simulink model "mariner_NNcont"  (R2018b)
settings: Solver=FixedStepAuto  StartTime=0.0  StopTime=600  FixedStep=0.1  RelTol=1e-3
libraries: neural x50, simulink x1
(part 2 of 2)

== system mariner_NNcont/Controller/NN controller (w.o process) 2 inputs/Layer 3/LW{3,2} ==
  "ad{3,2}" : Inport  PortDimensions=10
      mask Display: e = 0.06;c1 = [120 230 180]/255;c2 = ([120 230 180]+0)/(256+128);c3 = ([120 230 180]+128)/(256+128);patch([0 1 1 0],[0 0 1 1],c1);patch([0 1 1 1-e 1-e 0+e],[0 0 1 1-e 0+e 0+e],c2);patch([0 0 1 1-e 0+e 0+e],[0 1 1 1-e 1-e 0+e],c3);plot([0 1 1 0 0],[0 0 1 1 0]);
  "IW{3,2}(1,:)'" : Constant  Value=[-0.48696402852144660133859588313498534262180328369140625;-0.84681627945538029411665092993644066154956817626953125;0;0;1.0152212048569406732667630421929061412811279296875;0;0;0.89789896717366257661296913283877074718475341796875;0.1672600396616808204885984423526679165661334991455078125;0]
      mask Display: e = 0.06;c1 = [120 150 230]/255;c2 = ([120 150 230]+0)/383;c3 = ([120 150 230]+128)/383;patch([0 1 1 0],[0 0 1 1],c1);patch([0 1 1 1-e 1-e 0+e],[0 0 1 1-e 0+e 0+e],c2);patch([0 0 1 1-e 0+e 0+e],[0 1 1 1-e 1-e 0+e],c3);plot([0 1 1 0 0],[0 0 1 1 0]);disp('weights');
  Mux : Mux  Inputs=1
      mask Display: e = 0.06;c1 = [120 150 230]/255;c2 = ([120 150 230]+0)/383;c3 = ([120 150 230]+128)/383;patch([0 1 1 0],[0 0 1 1],c1);patch([0 1 1 1-e 1-e 0+e],[0 0 1 1-e 0+e 0+e],c2);patch([0 0 1 1-e 0+e 0+e],[0 1 1 1-e 1-e 0+e],c3);plot([0 1 1 0 0],[0 0 1 1 0]);disp('Mux');
  dotprod1 : neural/Weight Functions/dotprod
  "lz{3,2}" : Outport
      mask Display: e = 0.06;c1 = [120 230 180]/255;c2 = ([120 230 180]+0)/(256+128);c3 = ([120 230 180]+128)/(256+128);patch([0 1 1 0],[0 0 1 1],c1);patch([0 1 1 1-e 1-e 0+e],[0 0 1 1-e 0+e 0+e],c2);patch([0 0 1 1-e 0+e 0+e],[0 1 1 1-e 1-e 0+e],c3);plot([0 1 1 0 0],[0 0 1 1 0]);
  wires:
  Mux/1 -> "lz{3,2}"/1
  dotprod1/1 -> Mux/1
  "ad{3,2}"/1 -> dotprod1/2
  "IW{3,2}(1,:)'"/1 -> dotprod1/1

== system mariner_NNcont/Controller/NN controller (w//o process) 3 inputs/Layer 1/Delays 1 ==
  "p{1}" : Inport  PortDimensions=3
      mask Display: e = 0.06;c1 = [120 230 180]/255;c2 = ([120 230 180]+0)/(256+128);c3 = ([120 230 180]+128)/(256+128);patch([0 1 1 0],[0 0 1 1],c1);patch([0 1 1 1-e 1-e 0+e],[0 0 1 1-e 0+e 0+e],c2);patch([0 0 1 1-e 0+e 0+e],[0 1 1 1-e 1-e 0+e],c3);plot([0 1 1 0 0],[0 0 1 1 0]);
  mux : Mux  Inputs=1
      mask Display: e = 0.06;c1 = [120 150 230]/255;c2 = ([120 150 230]+0)/383;c3 = ([120 150 230]+128)/383;patch([0 1 1 0],[0 0 1 1],c1);patch([0 1 1 1-e 1-e 0+e],[0 0 1 1-e 0+e 0+e],c2);patch([0 0 1 1-e 0+e 0+e],[0 1 1 1-e 1-e 0+e],c3);plot([0 1 1 0 0],[0 0 1 1 0]);disp('Mux')
  "pd{1,1}" : Outport
      mask Display: e = 0.06;c1 = [120 230 180]/255;c2 = ([120 230 180]+0)/(256+128);c3 = ([120 230 180]+128)/(256+128);patch([0 1 1 0],[0 0 1 1],c1);patch([0 1 1 1-e 1-e 0+e],[0 0 1 1-e 0+e 0+e],c2);patch([0 0 1 1-e 0+e 0+e],[0 1 1 1-e 1-e 0+e],c3);plot([0 1 1 0 0],[0 0 1 1 0]);
  wires:
  mux/1 -> "pd{1,1}"/1
  "p{1}"/1 -> mux/1

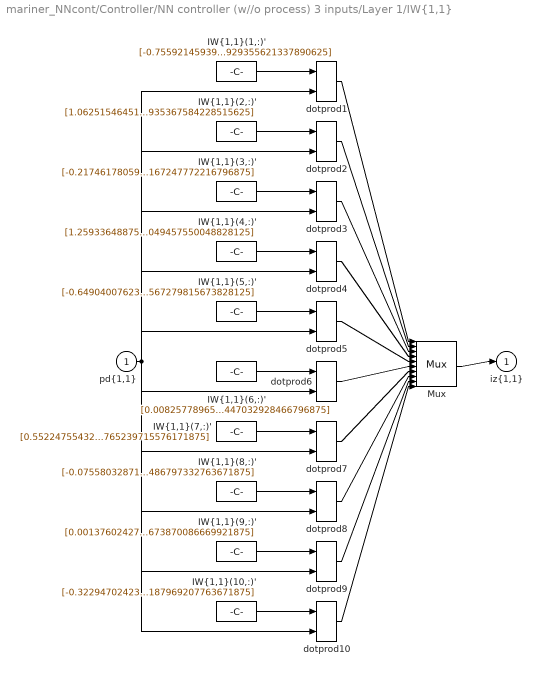
== system mariner_NNcont/Controller/NN controller (w//o process) 3 inputs/Layer 1/IW{1,1} ==
  "pd{1,1}" : Inport  PortDimensions=3
      mask Display: e = 0.06;c1 = [120 230 180]/255;c2 = ([120 230 180]+0)/(256+128);c3 = ([120 230 180]+128)/(256+128);patch([0 1 1 0],[0 0 1 1],c1);patch([0 1 1 1-e 1-e 0+e],[0 0 1 1-e 0+e 0+e],c2);patch([0 0 1 1-e 0+e 0+e],[0 1 1 1-e 1-e 0+e],c3);plot([0 1 1 0 0],[0 0 1 1 0]);
  "IW{1,1}(1,:)'" : Constant  Value=[-0.7559214593946765869958426264929585158824920654296875;-0.0246645007907288528470335364772836328484117984771728515625;0.031250654238925125449899411478327238000929355621337890625]
      mask Display: e = 0.06;c1 = [120 150 230]/255;c2 = ([120 150 230]+0)/383;c3 = ([120 150 230]+128)/383;patch([0 1 1 0],[0 0 1 1],c1);patch([0 1 1 1-e 1-e 0+e],[0 0 1 1-e 0+e 0+e],c2);patch([0 0 1 1-e 0+e 0+e],[0 1 1 1-e 1-e 0+e],c3);plot([0 1 1 0 0],[0 0 1 1 0]);disp('Weights');
  "IW{1,1}(10,:)'" : Constant  Value=[-0.32294702423027465965077453802223317325115203857421875;-0.1071172496029534626504897687482298351824283599853515625;0.0984226273448558230949601011161576025187969207763671875]
      mask Display: e = 0.06;c1 = [120 150 230]/255;c2 = ([120 150 230]+0)/383;c3 = ([120 150 230]+128)/383;patch([0 1 1 0],[0 0 1 1],c1);patch([0 1 1 1-e 1-e 0+e],[0 0 1 1-e 0+e 0+e],c2);patch([0 0 1 1-e 0+e 0+e],[0 1 1 1-e 1-e 0+e],c3);plot([0 1 1 0 0],[0 0 1 1 0]);disp('Weights');
  "IW{1,1}(2,:)'" : Constant  Value=[1.0625154645189052171616594932856969535350799560546875;0.1231458876428332960273337448597885668277740478515625;-0.12089326066373841384038456681082607246935367584228515625]
      mask Display: e = 0.06;c1 = [120 150 230]/255;c2 = ([120 150 230]+0)/383;c3 = ([120 150 230]+128)/383;patch([0 1 1 0],[0 0 1 1],c1);patch([0 1 1 1-e 1-e 0+e],[0 0 1 1-e 0+e 0+e],c2);patch([0 0 1 1-e 0+e 0+e],[0 1 1 1-e 1-e 0+e],c3);plot([0 1 1 0 0],[0 0 1 1 0]);disp('Weights');
  "IW{1,1}(3,:)'" : Constant  Value=[-0.2174617805911333856538902864485862664878368377685546875;-0.05222802197034777382800285749908653087913990020751953125;0.0405135495877011198029293836953002028167247772216796875]
      mask Display: e = 0.06;c1 = [120 150 230]/255;c2 = ([120 150 230]+0)/383;c3 = ([120 150 230]+128)/383;patch([0 1 1 0],[0 0 1 1],c1);patch([0 1 1 1-e 1-e 0+e],[0 0 1 1-e 0+e 0+e],c2);patch([0 0 1 1-e 0+e 0+e],[0 1 1 1-e 1-e 0+e],c3);plot([0 1 1 0 0],[0 0 1 1 0]);disp('Weights');
  "IW{1,1}(4,:)'" : Constant  Value=[1.259336488753712846033749883645214140415191650390625;0.12858048113142583890322612205636687576770782470703125;-0.12856053982931670010003699644585140049457550048828125]
      mask Display: e = 0.06;c1 = [120 150 230]/255;c2 = ([120 150 230]+0)/383;c3 = ([120 150 230]+128)/383;patch([0 1 1 0],[0 0 1 1],c1);patch([0 1 1 1-e 1-e 0+e],[0 0 1 1-e 0+e 0+e],c2);patch([0 0 1 1-e 0+e 0+e],[0 1 1 1-e 1-e 0+e],c3);plot([0 1 1 0 0],[0 0 1 1 0]);disp('Weights');
  "IW{1,1}(5,:)'" : Constant  Value=[-0.64904007623710613383849477031617425382137298583984375;-0.07309425860026873278396664090905687771737575531005859375;0.07976020263064671766972679733953555114567279815673828125]
      mask Display: e = 0.06;c1 = [120 150 230]/255;c2 = ([120 150 230]+0)/383;c3 = ([120 150 230]+128)/383;patch([0 1 1 0],[0 0 1 1],c1);patch([0 1 1 1-e 1-e 0+e],[0 0 1 1-e 0+e 0+e],c2);patch([0 0 1 1-e 0+e 0+e],[0 1 1 1-e 1-e 0+e],c3);plot([0 1 1 0 0],[0 0 1 1 0]);disp('Weights');
  "IW{1,1}(6,:)'" : Constant  Value=[0.0082577896598646817472033632157035754062235355377197265625;-0.043198240899638508383251433997429558075964450836181640625;0.038175683250024732007243954967634635977447032928466796875]
      mask Display: e = 0.06;c1 = [120 150 230]/255;c2 = ([120 150 230]+0)/383;c3 = ([120 150 230]+128)/383;patch([0 1 1 0],[0 0 1 1],c1);patch([0 1 1 1-e 1-e 0+e],[0 0 1 1-e 0+e 0+e],c2);patch([0 0 1 1-e 0+e 0+e],[0 1 1 1-e 1-e 0+e],c3);plot([0 1 1 0 0],[0 0 1 1 0]);disp('Weights');
  "IW{1,1}(7,:)'" : Constant  Value=[0.5522475543267157949145484963082708418369293212890625;0.038102250776124939324329687906356411986052989959716796875;-0.034686212621672755929136400254719774238765239715576171875]
      mask Display: e = 0.06;c1 = [120 150 230]/255;c2 = ([120 150 230]+0)/383;c3 = ([120 150 230]+128)/383;patch([0 1 1 0],[0 0 1 1],c1);patch([0 1 1 1-e 1-e 0+e],[0 0 1 1-e 0+e 0+e],c2);patch([0 0 1 1-e 0+e 0+e],[0 1 1 1-e 1-e 0+e],c3);plot([0 1 1 0 0],[0 0 1 1 0]);disp('Weights');
  "IW{1,1}(8,:)'" : Constant  Value=[-0.075580328717062272847471149361808784306049346923828125;-0.1184719143490288451037173445001826621592044830322265625;0.09404446170240236824167112672512303106486797332763671875]
      mask Display: e = 0.06;c1 = [120 150 230]/255;c2 = ([120 150 230]+0)/383;c3 = ([120 150 230]+128)/383;patch([0 1 1 0],[0 0 1 1],c1);patch([0 1 1 1-e 1-e 0+e],[0 0 1 1-e 0+e 0+e],c2);patch([0 0 1 1-e 0+e 0+e],[0 1 1 1-e 1-e 0+e],c3);plot([0 1 1 0 0],[0 0 1 1 0]);disp('Weights');
  "IW{1,1}(9,:)'" : Constant  Value=[0.0013760242756342658428103664647323967074044048786163330078125;-0.00880586545902399542296024037568713538348674774169921875;-0.0023602613359520771378619041769297837163321673870086669921875]
      mask Display: e = 0.06;c1 = [120 150 230]/255;c2 = ([120 150 230]+0)/383;c3 = ([120 150 230]+128)/383;patch([0 1 1 0],[0 0 1 1],c1);patch([0 1 1 1-e 1-e 0+e],[0 0 1 1-e 0+e 0+e],c2);patch([0 0 1 1-e 0+e 0+e],[0 1 1 1-e 1-e 0+e],c3);plot([0 1 1 0 0],[0 0 1 1 0]);disp('Weights');
  Mux : Mux  Inputs=10
      mask Display: e = 0.06;c1 = [120 150 230]/255;c2 = ([120 150 230]+0)/383;c3 = ([120 150 230]+128)/383;patch([0 1 1 0],[0 0 1 1],c1);patch([0 1 1 1-e 1-e 0+e],[0 0 1 1-e 0+e 0+e],c2);patch([0 0 1 1-e 0+e 0+e],[0 1 1 1-e 1-e 0+e],c3);plot([0 1 1 0 0],[0 0 1 1 0]);disp('Mux');
  dotprod{1..10} (10 alike) : neural/Weight Functions/dotprod
  "iz{1,1}" : Outport
      mask Display: e = 0.06;c1 = [120 230 180]/255;c2 = ([120 230 180]+0)/(256+128);c3 = ([120 230 180]+128)/(256+128);patch([0 1 1 0],[0 0 1 1],c1);patch([0 1 1 1-e 1-e 0+e],[0 0 1 1-e 0+e 0+e],c2);patch([0 0 1 1-e 0+e 0+e],[0 1 1 1-e 1-e 0+e],c3);plot([0 1 1 0 0],[0 0 1 1 0]);
  wires:
  Mux/1 -> "iz{1,1}"/1
  dotprod10/1 -> Mux/10
  "IW{1,1}(10,:)'"/1 -> dotprod10/1
  dotprod9/1 -> Mux/9
  "IW{1,1}(9,:)'"/1 -> dotprod9/1
  dotprod8/1 -> Mux/8
  "IW{1,1}(8,:)'"/1 -> dotprod8/1
  dotprod7/1 -> Mux/7
  "IW{1,1}(7,:)'"/1 -> dotprod7/1
  dotprod6/1 -> Mux/6
  "IW{1,1}(6,:)'"/1 -> dotprod6/1
  dotprod5/1 -> Mux/5
  "IW{1,1}(5,:)'"/1 -> dotprod5/1
  dotprod4/1 -> Mux/4
  "IW{1,1}(4,:)'"/1 -> dotprod4/1
  dotprod3/1 -> Mux/3
  "IW{1,1}(3,:)'"/1 -> dotprod3/1
  dotprod2/1 -> Mux/2
  "IW{1,1}(2,:)'"/1 -> dotprod2/1
  dotprod1/1 -> Mux/1
  "pd{1,1}"/1 -> dotprod10/2, dotprod9/2, dotprod8/2, dotprod7/2, dotprod6/2, dotprod5/2, dotprod4/2, dotprod3/2, dotprod2/2, dotprod1/2
  "IW{1,1}(1,:)'"/1 -> dotprod1/1

== system mariner_NNcont/Controller/NN controller (w//o process) 3 inputs/Layer 2/Delays 1 ==
  "p{2}" : Inport  PortDimensions=10
      mask Display: e = 0.06;c1 = [120 230 180]/255;c2 = ([120 230 180]+0)/(256+128);c3 = ([120 230 180]+128)/(256+128);patch([0 1 1 0],[0 0 1 1],c1);patch([0 1 1 1-e 1-e 0+e],[0 0 1 1-e 0+e 0+e],c2);patch([0 0 1 1-e 0+e 0+e],[0 1 1 1-e 1-e 0+e],c3);plot([0 1 1 0 0],[0 0 1 1 0]);
  mux : Mux  Inputs=1
      mask Display: e = 0.06;c1 = [120 150 230]/255;c2 = ([120 150 230]+0)/383;c3 = ([120 150 230]+128)/383;patch([0 1 1 0],[0 0 1 1],c1);patch([0 1 1 1-e 1-e 0+e],[0 0 1 1-e 0+e 0+e],c2);patch([0 0 1 1-e 0+e 0+e],[0 1 1 1-e 1-e 0+e],c3);plot([0 1 1 0 0],[0 0 1 1 0]);disp('Mux')
  "pd{2,1}" : Outport
      mask Display: e = 0.06;c1 = [120 230 180]/255;c2 = ([120 230 180]+0)/(256+128);c3 = ([120 230 180]+128)/(256+128);patch([0 1 1 0],[0 0 1 1],c1);patch([0 1 1 1-e 1-e 0+e],[0 0 1 1-e 0+e 0+e],c2);patch([0 0 1 1-e 0+e 0+e],[0 1 1 1-e 1-e 0+e],c3);plot([0 1 1 0 0],[0 0 1 1 0]);
  wires:
  mux/1 -> "pd{2,1}"/1
  "p{2}"/1 -> mux/1

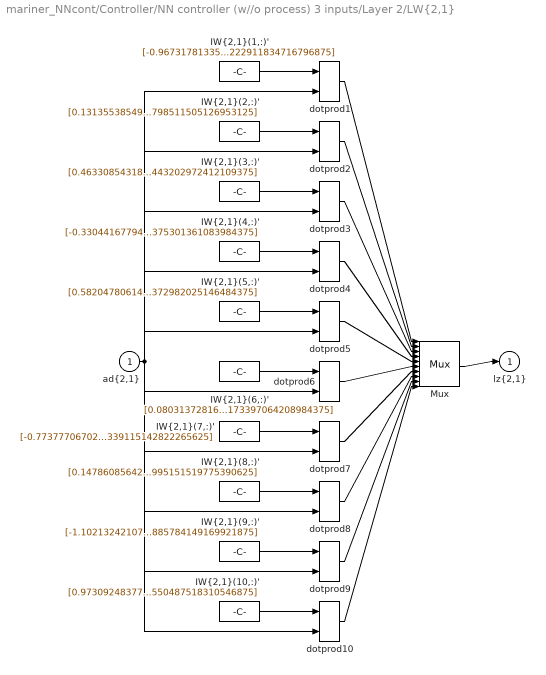
== system mariner_NNcont/Controller/NN controller (w//o process) 3 inputs/Layer 2/LW{2,1} ==
  "ad{2,1}" : Inport  PortDimensions=10
      mask Display: e = 0.06;c1 = [120 230 180]/255;c2 = ([120 230 180]+0)/(256+128);c3 = ([120 230 180]+128)/(256+128);patch([0 1 1 0],[0 0 1 1],c1);patch([0 1 1 1-e 1-e 0+e],[0 0 1 1-e 0+e 0+e],c2);patch([0 0 1 1-e 0+e 0+e],[0 1 1 1-e 1-e 0+e],c3);plot([0 1 1 0 0],[0 0 1 1 0]);
  "IW{2,1}(1,:)'" : Constant  Value=[-0.9673178133559503510952026772429235279560089111328125;0.53839778171147634200366383083746768534183502197265625;-0.722317642025362971480717533268034458160400390625;0.8553552777126747219682556533371098339557647705078125;0.275878338813815293661946270731277763843536376953125;-0.02755546810020788328632335151269217021763324737548828125;0.82237984032601907369297578043187968432903289794921875;-0.2547472202517508943486745920381508767604827880859375;-0.61557536337765605960470338686718605458736419677734375;0.153664159931131638625600999148446135222911834716796875]
      mask Display: e = 0.06;c1 = [120 150 230]/255;c2 = ([120 150 230]+0)/383;c3 = ([120 150 230]+128)/383;patch([0 1 1 0],[0 0 1 1],c1);patch([0 1 1 1-e 1-e 0+e],[0 0 1 1-e 0+e 0+e],c2);patch([0 0 1 1-e 0+e 0+e],[0 1 1 1-e 1-e 0+e],c3);plot([0 1 1 0 0],[0 0 1 1 0]);disp('weights');
  "IW{2,1}(10,:)'" : Constant  Value=[0.97309248377746315750158601076691411435604095458984375;-0.845856659992735959718856975086964666843414306640625;0.0295346903368784718946216116819414310157299041748046875;-1.1110911960074727478087197596323676407337188720703125;0.3060928624502607942048371114651672542095184326171875;-0.026387217399169611564690995919590932317078113555908203125;-0.554579983764879269614311851910315454006195068359375;-0.7959887047101454893294203429832123219966888427734375;-0.53675247865637409905303911727969534695148468017578125;-0.30786197281541471948429489202680997550487518310546875]
      mask Display: e = 0.06;c1 = [120 150 230]/255;c2 = ([120 150 230]+0)/383;c3 = ([120 150 230]+128)/383;patch([0 1 1 0],[0 0 1 1],c1);patch([0 1 1 1-e 1-e 0+e],[0 0 1 1-e 0+e 0+e],c2);patch([0 0 1 1-e 0+e 0+e],[0 1 1 1-e 1-e 0+e],c3);plot([0 1 1 0 0],[0 0 1 1 0]);disp('weights');
  "IW{2,1}(2,:)'" : Constant  Value=[0.1313553854999522096935749004842364229261875152587890625;-0.79774829886561471337103057521744631230831146240234375;-0.286014502405725845601835999332251958549022674560546875;1.1879656245342637976847299796645529568195343017578125;-0.70701622775883998794910212382092140614986419677734375;0.1677083387146580395477002412008005194365978240966796875;-0.46969451886407587171134991876897402107715606689453125;-0.138127570352924611274403332572546787559986114501953125;-0.43525645097113885295669888364500366151332855224609375;0.050289888408718404211317221097488072700798511505126953125]
      mask Display: e = 0.06;c1 = [120 150 230]/255;c2 = ([120 150 230]+0)/383;c3 = ([120 150 230]+128)/383;patch([0 1 1 0],[0 0 1 1],c1);patch([0 1 1 1-e 1-e 0+e],[0 0 1 1-e 0+e 0+e],c2);patch([0 0 1 1-e 0+e 0+e],[0 1 1 1-e 1-e 0+e],c3);plot([0 1 1 0 0],[0 0 1 1 0]);disp('weights');
  "IW{2,1}(3,:)'" : Constant  Value=[0.463308543185886156923203316182480193674564361572265625;0.01474050328529204374750083417211499181576073169708251953125;0.5708458173938455448848117157467640936374664306640625;-0.36304390338556735695618726822431199252605438232421875;0.03802927902901009904468310196534730494022369384765625;0.8688905579410917123794888539123348891735076904296875;-0.368022670402931073585506283052382059395313262939453125;1.078571025995817223019912489689886569976806640625;-0.42042514591632340614779650422860868275165557861328125;0.449357619793621321235832510865293443202972412109375]
      mask Display: e = 0.06;c1 = [120 150 230]/255;c2 = ([120 150 230]+0)/383;c3 = ([120 150 230]+128)/383;patch([0 1 1 0],[0 0 1 1],c1);patch([0 1 1 1-e 1-e 0+e],[0 0 1 1-e 0+e 0+e],c2);patch([0 0 1 1-e 0+e 0+e],[0 1 1 1-e 1-e 0+e],c3);plot([0 1 1 0 0],[0 0 1 1 0]);disp('weights');
  "IW{2,1}(4,:)'" : Constant  Value=[-0.330441677946859357906106424707104451954364776611328125;0.9398932320279040908417300670407712459564208984375;0.024098708014007048927584975217541796155273914337158203125;0.4618698985408240531569390441291034221649169921875;-1.1397682984094237301775365267531014978885650634765625;0.860210379926586110599373569129966199398040771484375;-0.17513721026530471025495216963463462889194488525390625;-0.410569653732319128636163441115058958530426025390625;-0.5560344839229272029257344911457039415836334228515625;-0.308418252656767977182283857473521493375301361083984375]
      mask Display: e = 0.06;c1 = [120 150 230]/255;c2 = ([120 150 230]+0)/383;c3 = ([120 150 230]+128)/383;patch([0 1 1 0],[0 0 1 1],c1);patch([0 1 1 1-e 1-e 0+e],[0 0 1 1-e 0+e 0+e],c2);patch([0 0 1 1-e 0+e 0+e],[0 1 1 1-e 1-e 0+e],c3);plot([0 1 1 0 0],[0 0 1 1 0]);disp('weights');
  "IW{2,1}(5,:)'" : Constant  Value=[0.58204780614894213730536876028054393827915191650390625;0.6967907615499668860792326086084358394145965576171875;0.99667255359175188633713560193427838385105133056640625;-0.699431723040012887082639281288720667362213134765625;-0.46866769281885722886471512538264505565166473388671875;-0.140751847389412765298999374863342382013797760009765625;0.12716603274524984623639056735555641353130340576171875;0.62879100504427842821542071760632097721099853515625;0.18062992316508286183562859150697477161884307861328125;0.3404346384178766893313650143682025372982025146484375]
      mask Display: e = 0.06;c1 = [120 150 230]/255;c2 = ([120 150 230]+0)/383;c3 = ([120 150 230]+128)/383;patch([0 1 1 0],[0 0 1 1],c1);patch([0 1 1 1-e 1-e 0+e],[0 0 1 1-e 0+e 0+e],c2);patch([0 0 1 1-e 0+e 0+e],[0 1 1 1-e 1-e 0+e],c3);plot([0 1 1 0 0],[0 0 1 1 0]);disp('weights');
  "IW{2,1}(6,:)'" : Constant  Value=[0.08031372816249911228414504194006440229713916778564453125;-0.297973938059601428651745891329483129084110260009765625;0.64300070459735680916679712026962079107761383056640625;0.53040993310285677875270948788966052234172821044921875;-0.79049086677915136878169732881360687315464019775390625;0.0832509692935996803431208945767139084637165069580078125;0.718295773451751440319412722601555287837982177734375;0.2364318776000905175660449231145321391522884368896484375;-0.8074693176251519499686537528759799897670745849609375;-0.80866490504699528596432855920284055173397064208984375]
      mask Display: e = 0.06;c1 = [120 150 230]/255;c2 = ([120 150 230]+0)/383;c3 = ([120 150 230]+128)/383;patch([0 1 1 0],[0 0 1 1],c1);patch([0 1 1 1-e 1-e 0+e],[0 0 1 1-e 0+e 0+e],c2);patch([0 0 1 1-e 0+e 0+e],[0 1 1 1-e 1-e 0+e],c3);plot([0 1 1 0 0],[0 0 1 1 0]);disp('weights');
  "IW{2,1}(7,:)'" : Constant  Value=[-0.77377706702885273859493509007734246551990509033203125;0.376757424003904883846871598507277667522430419921875;-0.19997543976920895136828448812593705952167510986328125;0.70509502994817807586258595620165579020977020263671875;0.06363014764948270174382827235604054294526576995849609375;0.70247114849747216425157603225670754909515380859375;-0.57831088496463889381260514710447750985622406005859375;-0.2346865136461891709895866142687737010419368743896484375;0.312603908634070337679844442391186021268367767333984375;-0.91858990863328193743342353627667762339115142822265625]
      mask Display: e = 0.06;c1 = [120 150 230]/255;c2 = ([120 150 230]+0)/383;c3 = ([120 150 230]+128)/383;patch([0 1 1 0],[0 0 1 1],c1);patch([0 1 1 1-e 1-e 0+e],[0 0 1 1-e 0+e 0+e],c2);patch([0 0 1 1-e 0+e 0+e],[0 1 1 1-e 1-e 0+e],c3);plot([0 1 1 0 0],[0 0 1 1 0]);disp('weights');
  "IW{2,1}(8,:)'" : Constant  Value=[0.1478608564296591543207881613852805458009243011474609375;0.664531605347525644589268267736770212650299072265625;-0.441801587802395701043423059672932140529155731201171875;0.69565887282337224295503119719796814024448394775390625;0.00545381413161631113661886871568640344776213169097900390625;-0.92106408854380183992560660044546239078044891357421875;0.033361495389616628581830326538693043403327465057373046875;-0.79809310204494388063523047094349749386310577392578125;0.71885462226626295478837391783599741756916046142578125;-0.6699848944034219044851852231658995151519775390625]
      mask Display: e = 0.06;c1 = [120 150 230]/255;c2 = ([120 150 230]+0)/383;c3 = ([120 150 230]+128)/383;patch([0 1 1 0],[0 0 1 1],c1);patch([0 1 1 1-e 1-e 0+e],[0 0 1 1-e 0+e 0+e],c2);patch([0 0 1 1-e 0+e 0+e],[0 1 1 1-e 1-e 0+e],c3);plot([0 1 1 0 0],[0 0 1 1 0]);disp('weights');
  "IW{2,1}(9,:)'" : Constant  Value=[-1.102132421071642998100514887482859194278717041015625;-0.6682571900111622387186116611701436340808868408203125;0.292635550191234827810404794945497997105121612548828125;-0.2314539238324496983612021949738846160471439361572265625;0.57375985909356630454425385323702357709407806396484375;0.06759075797283618791677639592307968996465206146240234375;-0.52314955273553220838067545628291554749011993408203125;-0.2028998165833909295141523898564628325402736663818359375;0.66713933922251789088164741770015098154544830322265625;-0.460676733779915970057317053942824713885784149169921875]
      mask Display: e = 0.06;c1 = [120 150 230]/255;c2 = ([120 150 230]+0)/383;c3 = ([120 150 230]+128)/383;patch([0 1 1 0],[0 0 1 1],c1);patch([0 1 1 1-e 1-e 0+e],[0 0 1 1-e 0+e 0+e],c2);patch([0 0 1 1-e 0+e 0+e],[0 1 1 1-e 1-e 0+e],c3);plot([0 1 1 0 0],[0 0 1 1 0]);disp('weights');
  Mux : Mux  Inputs=10
      mask Display: e = 0.06;c1 = [120 150 230]/255;c2 = ([120 150 230]+0)/383;c3 = ([120 150 230]+128)/383;patch([0 1 1 0],[0 0 1 1],c1);patch([0 1 1 1-e 1-e 0+e],[0 0 1 1-e 0+e 0+e],c2);patch([0 0 1 1-e 0+e 0+e],[0 1 1 1-e 1-e 0+e],c3);plot([0 1 1 0 0],[0 0 1 1 0]);disp('Mux');
  dotprod{1..10} (10 alike) : neural/Weight Functions/dotprod
  "lz{2,1}" : Outport
      mask Display: e = 0.06;c1 = [120 230 180]/255;c2 = ([120 230 180]+0)/(256+128);c3 = ([120 230 180]+128)/(256+128);patch([0 1 1 0],[0 0 1 1],c1);patch([0 1 1 1-e 1-e 0+e],[0 0 1 1-e 0+e 0+e],c2);patch([0 0 1 1-e 0+e 0+e],[0 1 1 1-e 1-e 0+e],c3);plot([0 1 1 0 0],[0 0 1 1 0]);
  wires:
  Mux/1 -> "lz{2,1}"/1
  dotprod10/1 -> Mux/10
  "IW{2,1}(10,:)'"/1 -> dotprod10/1
  dotprod9/1 -> Mux/9
  "IW{2,1}(9,:)'"/1 -> dotprod9/1
  dotprod8/1 -> Mux/8
  "IW{2,1}(8,:)'"/1 -> dotprod8/1
  dotprod7/1 -> Mux/7
  "IW{2,1}(7,:)'"/1 -> dotprod7/1
  dotprod6/1 -> Mux/6
  "IW{2,1}(6,:)'"/1 -> dotprod6/1
  dotprod5/1 -> Mux/5
  "IW{2,1}(5,:)'"/1 -> dotprod5/1
  dotprod4/1 -> Mux/4
  "IW{2,1}(4,:)'"/1 -> dotprod4/1
  dotprod3/1 -> Mux/3
  "IW{2,1}(3,:)'"/1 -> dotprod3/1
  dotprod2/1 -> Mux/2
  "IW{2,1}(2,:)'"/1 -> dotprod2/1
  dotprod1/1 -> Mux/1
  "ad{2,1}"/1 -> dotprod10/2, dotprod9/2, dotprod8/2, dotprod7/2, dotprod6/2, dotprod5/2, dotprod4/2, dotprod3/2, dotprod2/2, dotprod1/2
  "IW{2,1}(1,:)'"/1 -> dotprod1/1

== system mariner_NNcont/Controller/NN controller (w//o process) 3 inputs/Layer 3/Delays 1 ==
  "p{3}" : Inport  PortDimensions=10
      mask Display: e = 0.06;c1 = [120 230 180]/255;c2 = ([120 230 180]+0)/(256+128);c3 = ([120 230 180]+128)/(256+128);patch([0 1 1 0],[0 0 1 1],c1);patch([0 1 1 1-e 1-e 0+e],[0 0 1 1-e 0+e 0+e],c2);patch([0 0 1 1-e 0+e 0+e],[0 1 1 1-e 1-e 0+e],c3);plot([0 1 1 0 0],[0 0 1 1 0]);
  mux : Mux  Inputs=1
      mask Display: e = 0.06;c1 = [120 150 230]/255;c2 = ([120 150 230]+0)/383;c3 = ([120 150 230]+128)/383;patch([0 1 1 0],[0 0 1 1],c1);patch([0 1 1 1-e 1-e 0+e],[0 0 1 1-e 0+e 0+e],c2);patch([0 0 1 1-e 0+e 0+e],[0 1 1 1-e 1-e 0+e],c3);plot([0 1 1 0 0],[0 0 1 1 0]);disp('Mux')
  "pd{3,2}" : Outport
      mask Display: e = 0.06;c1 = [120 230 180]/255;c2 = ([120 230 180]+0)/(256+128);c3 = ([120 230 180]+128)/(256+128);patch([0 1 1 0],[0 0 1 1],c1);patch([0 1 1 1-e 1-e 0+e],[0 0 1 1-e 0+e 0+e],c2);patch([0 0 1 1-e 0+e 0+e],[0 1 1 1-e 1-e 0+e],c3);plot([0 1 1 0 0],[0 0 1 1 0]);
  wires:
  mux/1 -> "pd{3,2}"/1
  "p{3}"/1 -> mux/1

== system mariner_NNcont/Controller/NN controller (w//o process) 3 inputs/Layer 3/LW{3,2} ==
  "ad{3,2}" : Inport  PortDimensions=10
      mask Display: e = 0.06;c1 = [120 230 180]/255;c2 = ([120 230 180]+0)/(256+128);c3 = ([120 230 180]+128)/(256+128);patch([0 1 1 0],[0 0 1 1],c1);patch([0 1 1 1-e 1-e 0+e],[0 0 1 1-e 0+e 0+e],c2);patch([0 0 1 1-e 0+e 0+e],[0 1 1 1-e 1-e 0+e],c3);plot([0 1 1 0 0],[0 0 1 1 0]);
  "IW{3,2}(1,:)'" : Constant  Value=[-0.73149029744197668900795861190999858081340789794921875;0;0;-0.84948708100111236518614532542414963245391845703125;0;-0.437042300450375176268380528199486434459686279296875;0;-0.66202787718184818999134222394786775112152099609375;0;1.1687904609959163249044422627775929868221282958984375]
      mask Display: e = 0.06;c1 = [120 150 230]/255;c2 = ([120 150 230]+0)/383;c3 = ([120 150 230]+128)/383;patch([0 1 1 0],[0 0 1 1],c1);patch([0 1 1 1-e 1-e 0+e],[0 0 1 1-e 0+e 0+e],c2);patch([0 0 1 1-e 0+e 0+e],[0 1 1 1-e 1-e 0+e],c3);plot([0 1 1 0 0],[0 0 1 1 0]);disp('weights');
  Mux : Mux  Inputs=1
      mask Display: e = 0.06;c1 = [120 150 230]/255;c2 = ([120 150 230]+0)/383;c3 = ([120 150 230]+128)/383;patch([0 1 1 0],[0 0 1 1],c1);patch([0 1 1 1-e 1-e 0+e],[0 0 1 1-e 0+e 0+e],c2);patch([0 0 1 1-e 0+e 0+e],[0 1 1 1-e 1-e 0+e],c3);plot([0 1 1 0 0],[0 0 1 1 0]);disp('Mux');
  dotprod1 : neural/Weight Functions/dotprod
  "lz{3,2}" : Outport
      mask Display: e = 0.06;c1 = [120 230 180]/255;c2 = ([120 230 180]+0)/(256+128);c3 = ([120 230 180]+128)/(256+128);patch([0 1 1 0],[0 0 1 1],c1);patch([0 1 1 1-e 1-e 0+e],[0 0 1 1-e 0+e 0+e],c2);patch([0 0 1 1-e 0+e 0+e],[0 1 1 1-e 1-e 0+e],c3);plot([0 1 1 0 0],[0 0 1 1 0]);
  wires:
  Mux/1 -> "lz{3,2}"/1
  dotprod1/1 -> Mux/1
  "ad{3,2}"/1 -> dotprod1/2
  "IW{3,2}(1,:)'"/1 -> dotprod1/1

== matlab function mariner_NNcont/MATLAB Function1 ==
  data: xdot input; xnext output; x input; h input
function xnext = euler2(xdot,x,h)
% EULER2  Integrate a system of ordinary differential equations using 
%	  Euler's 2nd-order method.
%
% xnext = euler2(xdot,x,h)
%
% xdot  - dx/dt(k) = f(x(k)
% x     - x(k)
% xnext - x(k+1)
% h     - step size
%
% Author:   Thor I. Fossen
% Date:     14th June 2001
% Revisions: 

xnext = x + h*xdot;

== matlab function mariner_NNcont/MATLAB Function ==
  data: x input; xdot output; ui input
function xdot   = mariner(x,ui)
% [xdot,U] = mariner(x,ui) returns the speed U in m/s (optionally) and the 
% time derivative of the state vector: x = [ u v r x y psi delta n ]'  for
% the Mariner class vessel L = 160.93 m, where
%
% u     = pertubed surge velocity about Uo (m/s)
% v     = pertubed sway velocity about zero (m/s)
% r     = pertubed yaw velocity about zero (rad/s)
% x     = position in x-direction (m)
% y     = position in y-direction (m)
% psi   = pertubed yaw angle about zero (rad)
% delta = actual rudder angle (rad)
%
% The inputs are :
% 
% ui    = commanded rudder angle (rad)
% U0    = nominal speed (optionally). Default value is U0 = 7.7175 m/s = 15 knots.
%
% Reference: M.S. Chislett and J. Stroem-Tejsen (1965). Planar Motion Mechanism Tests 
%            and Full-Scale Steering and Maneuvering Predictions for a Mariner Class Vessel,
%            Technical Report Hy-5, Hydro- and Aerodynamics Laboratory, Lyngby, Denmark.
% 
% Author:    Trygve Lauvdal
% Date:      12th May 1994
% Revisions: 19th July 2001 (Thor I. Fossen): added input/ouput U0 and U, changed order of x-vector
%            20th July 2001 (Thor I. Fossen): replaced inertia matrix with correct values
%            11th July 2003 (Thor I. Fossen): max rudder is changed from 30 deg to 40
%                            deg to satisfy IMO regulations for 35 deg rudder execute

% Check of input and state dimensions
if (length(x)  ~= 7),error('x-vector must have dimension 7 !'); end
if (length(ui) ~= 1),error('ui must be a scalar input!'); end
%if nargin==2, U0 = 7.7175; end

U0 = 7.7175;

% Normalization variables
L = 160.93;
U = sqrt((U0 + x(1))^2 + x(2)^2);

% Non-dimensional states and inputs
delta_c = -ui;   % delta_c = -ui such that positive delta_c -> positive r

u     = x(1)/U;   
v     = x(2)/U;  
r     = x(3)*L/U; 
psi   = x(6); 
delta = x(7); 

% Parameters, hydrodynamic derivatives and main dimensions
delta_max  = 40;           % max rudder angle      (deg)
Ddelta_max = 5;            % max rudder derivative (deg/s)

m  = 798e-5;
Iz = 39.2e-5;
xG = -0.023;

Xudot =  -42e-5;   Yvdot =  -748e-5;   Nvdot = 4.646e-5;
Xu    = -184e-5;   Yrdot =-9.354e-5;   Nrdot = -43.8e-5;
Xuu   = -110e-5;   Yv    = -1160e-5;   Nv    =  -264e-5;
Xuuu  = -215e-5;   Yr    =  -499e-5;   Nr    =  -166e-5;
Xvv   = -899e-5;   Yvvv  = -8078e-5;   Nvvv  =  1636e-5;
Xrr   =   18e-5;   Yvvr  = 15356e-5;   Nvvr  = -5483e-5;
Xdd   =  -95e-5;   Yvu   = -1160e-5;   Nvu   =  -264e-5;
Xudd  = -190e-5;   Yru   =  -499e-5;   Nru   =  -166e-5;
Xrv   =  798e-5;   Yd    =   278e-5;   Nd    =  -139e-5;
Xvd   =   93e-5;   Yddd  =   -90e-5;   Nddd  =    45e-5;
Xuvd  =   93e-5;   Yud   =   556e-5;   Nud   =  -278e-5;
                   Yuud  =   278e-5;   Nuud  =  -139e-5;
                   Yvdd  =    -4e-5;   Nvdd  =    13e-5;
                   Yvvd  =  1190e-5;   Nvvd  =  -489e-5;
                   Y0    =    -4e-5;   N0    =     3e-5;
                   Y0u   =    -8e-5;   N0u   =     6e-5;
                   Y0uu  =    -4e-5;   N0uu  =     3e-5;

% Masses and moments of inertia
m11 = m-Xudot;
m22 = m-Yvdot;
m23 = m*xG-Yrdot;
m32 = m*xG-Nvdot;
m33 = Iz-Nrdot;

% Rudder saturation and dynamics
if abs(delta_c) >= delta_max*pi/180,
   delta_c = sign(delta_c)*delta_max*pi/180;
end
delta_dot = delta_c - delta;
if abs(delta_dot) >= Ddelta_max*pi/180,
   delta_dot = sign(delta_dot)*Ddelta_max*pi/180;
end

% Forces and moments
X = Xu*u + Xuu*u^2 + Xuuu*u^3 + Xvv*v^2 + Xrr*r^2 + Xrv*r*v + Xdd*delta^2 +...
    Xudd*u*delta^2 + Xvd*v*delta + Xuvd*u*v*delta;

Y = Yv*v + Yr*r + Yvvv*v^3 + Yvvr*v^2*r + Yvu*v*u + Yru*r*u + Yd*delta + ...
    Yddd*delta^3 + Yud*u*delta + Yuud*u^2*delta + Yvdd*v*delta^2 + ...
    Yvvd*v^2*delta + (Y0 + Y0u*u + Y0uu*u^2);

N = Nv*v + Nr*r + Nvvv*v^3 + Nvvr*v^2*r + Nvu*v*u + Nru*r*u + Nd*delta + ...
    Nddd*delta^3 + Nud*u*delta + Nuud*u^2*delta + Nvdd*v*delta^2 + ...
    Nvvd*v^2*delta + (N0 + N0u*u + N0uu*u^2);

% Dimensional state derivative
detM22 = m22*m33-m23*m32;

xdot = [           X*(U^2/L)/m11
        -(-m33*Y+m23*N)*(U^2/L)/detM22
         (-m32*Y+m22*N)*(U^2/L^2)/detM22
           (cos(psi)*(U0/U+u)-sin(psi)*v)*U
           (sin(psi)*(U0/U+u)+cos(psi)*v)*U  
                    r*(U/L)
                    delta_dot                  ];

== stateflow chart mariner_NNcont/mariner ==
  settings: updateMethod=CONTINUOUS
  state mariner
    %% initialize values when entry
    en:
    L = 160.93;
    m = 798*10^-5;
    xG = -0.023;
    Iz = 39.2*10^-5;
    Xudot =  -42e-5;  Yvdot =  -748e-5;  Nvdot = 4.646e-5;
    Xu  = -184e-5;   Yrdot =-9.354e-5;   Nrdot = -43.8e-5;
    Xuu = -110e-5;   Yv = -1160e-5;   Nv =  -264e-5;
    Xuuu = -215e-5;   Yr =  -499e-5;   Nr =  -166e-5;
    Xvv = -899e-5;   Yvvv = -8078e-5;   Nvvv =  1636e-5;
    Xrr =   18e-5;   Yvvr = 15356e-5;   Nvvr = -5483e-5;
    Xdd =  -95e-5;   Yvu = -1160e-5;   Nvu =  -264e-5;
    Xudd = -190e-5;   Yru =  -499e-5;   Nru =  -166e-5;
    Xrv =  798e-5;   Yd  =   278e-5;   Nd =  -139e-5;
    Xvd =   93e-5;   Yddd  =   -90e-5;   Nddd =    45e-5;
    Xuvd =   93e-5;   Yud = 556e-5;   Nud =  -278e-5;
    Yuud =   278e-5;   Nuud  =  -139e-5;
    Yvdd  =    -4e-5;   Nvdd  = 13e-5;
    Yvvd  =  1190e-5;   Nvvd  = -489e-5;
    Y0 = -4e-5;   N0 =  3e-5;
    Y0u  =  -8e-5;   N0u = 6e-5;
    Y0uu =  -4e-5;   N0uu  =  3e-5;
    m11 = 798*10^-5 - (-42e-5);
    m22 = 798*10^-5 - ( -748e-5);
    m23 = 798*10^-5 * -0.023 - (-9.354e-5);
    m32 = 798*10^-5 * -0.023 - 4.646e-5;
    m33 = 39.2*10^-5 -  (-43.8e-5);
    %detM22 = m22*m33-m23*m32;
    %detM22 = ((798*10^-5 - ( -748e-5))*(39.2*10^-5 -  (-43.8e-5)) - (798*10^-5 * -0.023 - (-9.354e-5))*(798*10^-5 * -0.023 - 4.646e-5));
    delta_max = 40;
    Ddelta_max = 5;
    % u
    %Executing updates of system during simulation
    du:
    %delta_c = min(max(-ui,-delta_max*pi/180),delta_max*pi/180) ;
    %U = (sqrt((ui + u)^2 + v^2));
    %delta_do = (-ui - delta);
    %X = Xu*u/(sqrt((ui + u)^2 + v^2)) + Xuu*(u/(sqrt((ui + u)^2 + v^2)))^2 + Xuuu*(u/(sqrt((ui + u)^2 + v^2)))^3 + Xvv*(v/(sqrt((ui + u)^2 + v^2)))^2 + Xrr*(r*L/(sqrt((ui + u)^2 + v^2)))^2 + Xrv*(r*L/(sqrt((ui + u)^2 + v^2)))*(v/(sqrt((ui + u)^2 + v^2))) + Xdd*delta^2 +Xudd*(u/(sqrt((ui + u)^2 + v^2)))*delta^2 + Xvd*(v/(sqrt((ui + u)^2 + v^2)))*delta + Xuvd*(u/(sqrt((ui + u)^2 + v^2)))*(v/(sqrt((ui + u)^2 + v^2)))*delta;
    %Y = Yv*v + Yr*r + Yvvv*v^3 + Yvvr*v^2*r + Yvu*v*u + Yru*r*u + Yd*delta + Yddd*delta^3 + Yud*u*delta + Yuud*u^2*delta + Yvdd*v*delta^2 + Yvvd*v^2*delta + (Y0 + Y0u*u + Y0uu*u^2);
    %N = Nv*v + Nr*r + Nvvv*v^3 + Nvvr*v^2*r + Nvu*v*u + Nru*r*u + Nd*delta + Nddd*delta^3 + Nud*u*delta + Nuud*u^2*delta + Nvdd*v*delta^2 + Nvvd*v^2*delta + (N0 + N0u*u + N0uu*u^2);
    u_dot = (Xu*(u/(sqrt((ui + u)^2 + v^2))) + Xuu*(u/(sqrt((ui + u)^2 + v^2)))^2 + Xuuu*(u/(sqrt((ui + u)^2 + v^2)))^3 + Xvv*(v/(sqrt((ui + u)^2 + v^2)))^2 + Xrr*(r*L/(sqrt((ui + u)^2 + v^2)))^2 + Xrv*(r*L/(sqrt((ui + u)^2 + v^2)))*(v/(sqrt((ui + u)^2 + v^2))) + Xdd*delta^2 +Xudd*(u/(sqrt((ui + u)^2 + v^2)))*delta^2 + Xvd*(v/(sqrt((ui + u)^2 + v^2)))*delta + Xuvd*(u/(sqrt((ui + u)^2 + v^2)))*(v/(sqrt((ui + u)^2 + v^2)))*delta)*((sqrt((ui + u)^2 + v^2))^2 /L)/(798*10^-5 - (-42e-5));
    v_dot =  -(-(39.2*10^-5 -  (-43.8e-5))*(Yv*(v/(sqrt((ui + u)^2 + v^2))) + Yr*(r*L/(sqrt((ui + u)^2 + v^2))) + Yvvv*(v/(sqrt((ui + u)^2 + v^2)))^3 + Yvvr*(v/(sqrt((ui + u)^2 + v^2)))^2 * (r*L/(sqrt((ui + u)^2 + v^2))) + Yvu*(v/(sqrt((ui + u)^2 + v^2)))*(u/(sqrt((ui + u)^2 + v^2))) + Yru*(r*L/(sqrt((ui + u)^2 + v^2)))*(u/(sqrt((ui + u)^2 + v^2))) + Yd*delta + Yddd*delta^3 + Yud*(u/(sqrt((ui + u)^2 + v^2)))*delta + Yuud*(u/(sqrt((ui + u)^2 + v^2)))^2*delta + Yvdd*(v/(sqrt((ui + u)^2 + v^2)))*delta^2 + Yvvd*(v/(sqrt((ui + u)^2 + v^2)))^2*delta + (Y0 + Y0u*(u/(sqrt((ui + u)^2 + v^2))) + Y0uu*(u/(sqrt((ui + u)^2 + v^2)))^2))+(798*10^-5 * -0.023 - (-9.354e-5))*(Nv*(v/(sqrt((ui + u)^2 + v^2))) + Nr*(r*L/(sqrt((ui + u)^2 + v^2))) + Nvvv*(v/(sqrt((ui + u)^2 + v^2)))^3 + Nvvr*(v/(sqrt((ui + u)^2 + v^2)))^2*(r*L/(sqrt((ui + u)^2 + v^2))) + Nvu*(v/(sqrt((ui + u)^2 + v^2)))*(u/(sqrt((ui + u)^2 + v^2))) + Nru*(r*L/(sqrt((ui + u)^2 + v^2)))*(u/(sqrt((ui + u)^2 + v^2))) + Nd*delta + Nddd*delta^3 + Nud*(u/(sqrt((ui + u)^2 + v^2)))*delta + Nuud*(u/(sqrt((ui + u)^2 + v^2)))^2*delta + Nvdd*(v/(sqrt((ui + u)^2 + v^2)))*delta^2 + Nvvd*v^2*delta + (N0 + N0u*u + N0uu*u^2)))*((sqrt((ui + u)^2 + v^2))^2/L)/((798*10^-5 - ( -748e-5))*(39.2*10^-5 -  (-43.8e-5)) - (798*10^-5 * -0.023 - (-9.354e-5))*(798*10^-5 * -0.023 - 4.646e-5)) ;
    r_dot = (-(798*10^-5 * -0.023 - 4.646e-5)*(Yv*(v/(sqrt((ui + u)^2 + v^2))) + Yr*(r*L/(sqrt((ui + u)^2 + v^2))) + Yvvv*(v/(sqrt((ui + u)^2 + v^2)))^3 + Yvvr*(v/(sqrt((ui + u)^2 + v^2)))^2*(r*L/(sqrt((ui + u)^2 + v^2))) + Yvu*(v/(sqrt((ui + u)^2 + v^2)))*(u/(sqrt((ui + u)^2 + v^2))) + Yru*(r*L/(sqrt((ui + u)^2 + v^2)))*(u/(sqrt((ui + u)^2 + v^2))) + Yd*delta + Yddd*delta^3 + Yud*(u/(sqrt((ui + u)^2 + v^2)))*delta + Yuud*(u/(sqrt((ui + u)^2 + v^2)))^2*delta + Yvdd*(v/(sqrt((ui + u)^2 + v^2)))*delta^2 + Yvvd*(v/(sqrt((ui + u)^2 + v^2)))^2*delta + (Y0 + Y0u*(u/(sqrt((ui + u)^2 + v^2))) + Y0uu*(u/(sqrt((ui + u)^2 + v^2)))^2))+(798*10^-5 - ( -748e-5))*(Nv*(v/(sqrt((ui + u)^2 + v^2))) + Nr*(r*L/(sqrt((ui + u)^2 + v^2))) + Nvvv*(v/(sqrt((ui + u)^2 + v^2)))^3 + Nvvr*(v/(sqrt((ui + u)^2 + v^2)))^2*(r*L/(sqrt((ui + u)^2 + v^2))) + Nvu*(v/(sqrt((ui + u)^2 + v^2)))*(u/(sqrt((ui + u)^2 + v^2))) + Nru*(r*L/(sqrt((ui + u)^2 + v^2)))*(u/(sqrt((ui + u)^2 + v^2))) + Nd*delta + Nddd*delta^3 + Nud*(u/(sqrt((ui + u)^2 + v^2)))*delta + Nuud*(u/(sqrt((ui + u)^2 + v^2)))^2*delta + Nvdd*(v/(sqrt((ui + u)^2 + v^2)))*delta^2 + Nvvd*(v/(sqrt((ui + u)^2 + v^2)))^2*delta + (N0 + N0u*(u/(sqrt((ui + u)^2 + v^2))) + N0uu*(u/(sqrt((ui + u)^2 + v^2)))^2)))*((sqrt((ui + u)^2 + v^2))^2/L^2)/((798*10^-5 - ( -748e-5))*(39.2*10^-5 -  (-43.8e-5)) - (798*10^-5 * -0.023 - (-9.354e-5))*(798*10^-5 * -0.023 - 4.646e-5)) ;
    x_dot = (cos(psi)*(U0/(sqrt((ui + u)^2 + v^2))+(u/(sqrt((ui + u)^2 + v^2))))-sin(psi)*(v/(sqrt((ui + u)^2 + v^2))))*(sqrt((ui + u)^2 + v^2)) ;
    y_dot = (sin(psi)*(U0/(sqrt((ui + u)^2 + v^2))+(u/(sqrt((ui + u)^2 + v^2))))+cos(psi)*(v/(sqrt((ui + u)^2 + v^2))))*(sqrt((ui + u)^2 + v^2)) ;
    psi_dot = (r*L/(sqrt((ui + u)^2 + v^2)))*((sqrt((ui + u)^2 + v^2))/L);
    delta_dot = min(max(((min(max(-ui,-delta_max*pi/180),delta_max*pi/180)) - delta),-Ddelta_max*pi/180),Ddelta_max*pi/180) ;
    %% OUTPUTS
    u_out = u;
    v_out = v;
    r_out = r;
    x_out = x;
    y_out = y;
    psi_out = psi;
    delta_out = delta;
  (default) -> ? [order 1]
  (default) -> mariner [order 1] : {u = 0.01;
      | v = 0.01;
      | r = 0.01;
      | x = 0.01;
      | y = 0.01;
      | psi = 0.01;
      | delta = 0.01;}
  data: u_out output; v_out output; u local; ui input; v local; Nvdot local double; Iz local double; L local double; Yvdot local double; xG local double; m local double; Xudot local double; Xuu local double; Yv local double; Xuuu local double; Nrdot local double; Nv local double; Yr local double; Yrdot local double; Xu local double; Nr local double; Xrr local double; Xdd local double; Yvvv local double; Yvu local double; Nvvv local double; Yvvr local double; Nvvr local double; Xvv local double; Xvd local double; Yru local double; Nd local double; Nvu local double; Xudd local double; Nru local double; Yd local double; Xrv local double; Nvdd local double; Yud local double; Yuud local double; Xuvd local double; Yvdd local double; Nud local double; Nuud local double; Yddd local double; Nddd local double; Y0uu local double; N0uu local double; N0 local double; N0u local double; Y0 local double; Yvvd local double; Nvvd local double; Y0u local double; m11 local double; m32 local double; m22 local double; m23 local double; m33 local double; U0 input; r_out output; r local; psi local; x local; y local; delta local; Ddelta_max local double; delta_max local double; N local double; x_out output; y_out output; psi_out output double; delta_out output
  data u settings: updateMethod=SF_CONTINUOUS_TIME_DATA
  data v settings: updateMethod=SF_CONTINUOUS_TIME_DATA
  data r settings: updateMethod=SF_CONTINUOUS_TIME_DATA
  data psi settings: updateMethod=SF_CONTINUOUS_TIME_DATA
  data x settings: updateMethod=SF_CONTINUOUS_TIME_DATA
  data y settings: updateMethod=SF_CONTINUOUS_TIME_DATA
  data delta settings: updateMethod=SF_CONTINUOUS_TIME_DATA

== matlab function mariner_NNcont/Controller/Normalize ==
  data: u input; y output
function y = fcn(u)
max_r = 0.0029; min_r = -4.9078e-04;
max_psi = 0.1295; min_psi = 0;
y = zeros(3,1);
y(1) = (u(1) -min_r)/(max_r - min_r);% r
y(2) = (u(2) -min_psi)/(max_psi - min_psi);
y(3) = u(3);

== matlab function mariner_NNcont/Controller/denormalize ==
  data: u input; y output
function y = fcn(u)
max_delta = 0.0445; min_delta = -0.0779;
y = zeros(1,1);
y(1) = u(1)*(max_delta - min_delta)+min_delta;% r
